simulink model "dynamicANN"  (R2019b)
settings: Solver=VariableStepAuto  StartTime=0.0  StopTime=5  RelTol=1e-3
values from neighbouring files (symbols this model uses):
  a = 87.548e-3    (= 0.087548)    [main.m]
  b = 132.452e-3    (= 0.132452)    [main.m]
  d = 22.452e-3    (= 0.022452)    [main.m]
  delta = [dX 0 0 0; -dX 0 0 0; 0 dXdot 0 0; 0 -dXdot 0 0; 0 0 dY 0; 0 0 -dY 0; 0 0 0 dYdot; 0 0 0 -dYdot]    [dyn_coeff.m]    (also in main.m = 2.5e-05)
  F1 = mass*g-F2    (= 22.4020462598)    [main.m]
  F2 = a*mass*g/(a+b)    (= 14.8072837402)    [main.m]
  g = 9.8    [EOM.m]    (also in main.m = 9.81)
  Jd = 0.047331604    [main.m]
  Jp = 0.00075    [main.m]
  Kps = (Vmax-Vmin)/(Hmax-Hmin)    (= 1666.66666667)    [main.m]
  Ksv = 30    [main.m]
  mass = 3.793    [main.m]
  omega = operational_parameters(1)*2*pi/60    [CalculateLoadCapacity.m]    (also in main.m = 146.607657168)
  s = 30e-3    (= 0.03)    [main.m]    (also in nntrainingsetgen.m = size(XC))
  tau = 0.12    [main.m]
  taus = 0.00125    [main.m]
  Ts = 1/fs    (= 0.001)    [main.m]
libraries: neural x424, simulink x2
(part 8 of 10)

== system dynamicANN/ROTOR SYSTEM WITH ANN/B1NN/Layer 2/Delays 1 ==
  "p{2}" : Inport  PortDimensions=100
      mask Display: e = 0.06;c1 = [120 230 180]/255;c2 = ([120 230 180]+0)/(256+128);c3 = ([120 230 180]+128)/(256+128);patch([0 1 1 0],[0 0 1 1],c1);patch([0 1 1 1-e 1-e 0+e],[0 0 1 1-e 0+e 0+e],c2);patch([0 0 1 1-e 0+e 0+e],[0 1 1 1-e 1-e 0+e],c3);plot([0 1 1 0 0],[0 0 1 1 0]);
  mux : Mux  Inputs=1
      mask Display: e = 0.06;c1 = [120 150 230]/255;c2 = ([120 150 230]+0)/383;c3 = ([120 150 230]+128)/383;patch([0 1 1 0],[0 0 1 1],c1);patch([0 1 1 1-e 1-e 0+e],[0 0 1 1-e 0+e 0+e],c2);patch([0 0 1 1-e 0+e 0+e],[0 1 1 1-e 1-e 0+e],c3);plot([0 1 1 0 0],[0 0 1 1 0]);disp('Mux')
  "pd{2,1}" : Outport
      mask Display: e = 0.06;c1 = [120 230 180]/255;c2 = ([120 230 180]+0)/(256+128);c3 = ([120 230 180]+128)/(256+128);patch([0 1 1 0],[0 0 1 1],c1);patch([0 1 1 1-e 1-e 0+e],[0 0 1 1-e 0+e 0+e],c2);patch([0 0 1 1-e 0+e 0+e],[0 1 1 1-e 1-e 0+e],c3);plot([0 1 1 0 0],[0 0 1 1 0]);
  wires:
  "p{2}"/1 -> mux/1
  mux/1 -> "pd{2,1}"/1

== system dynamicANN/ROTOR SYSTEM WITH ANN/B1NN/Layer 2/LW{2,1} ==
  "ad{2,1}" : Inport  PortDimensions=100
      mask Display: e = 0.06;c1 = [120 230 180]/255;c2 = ([120 230 180]+0)/(256+128);c3 = ([120 230 180]+128)/(256+128);patch([0 1 1 0],[0 0 1 1],c1);patch([0 1 1 1-e 1-e 0+e],[0 0 1 1-e 0+e 0+e],c2);patch([0 0 1 1-e 0+e 0+e],[0 1 1 1-e 1-e 0+e],c3);plot([0 1 1 0 0],[0 0 1 1 0]);
  "IW{2,1}(1,:)'" : Constant  Value=[-4.30818797311500389923821785487234592437744140625;0.1752068552208518037449636040037148632109165191650390625;1.6512760960076289240561209226143546402454376220703125;-1.2668488416247047911866729918983764946460723876953125;-0.169916708135180172245526364349643699824810028076171875;2.667525323070837117711562314070761203765869140625;-3.694593268415584663699746670317836105823516845703125;-0.194624707793134177347127433677087537944316864013671875;3.883534816499157660274477166240103542804718017578125;-4.8924351217341808251148904673755168914794921875;0.16008181045926705987625382476835511624813079833984375;-4.0208522454679798130428025615401566028594970703125;2.81348078614510210826438196818344295024871826171875;-0.09088682268917881723613305666731321252882480621337890625;-0.361803208282506283399726498828385956585407257080078125;-2.550539713092682791995002844487316906452178955078125;0.06642984533116191858681531812180764973163604736328125;4.87354419159413776441169829922728240489959716796875;-3.155434137388119619771487123216502368450164794921875;0.04540205268647821978955647637121728621423244476318359375;3.523762597164889154299771689693443477153778076171875;1.2480467061721984833866372355259954929351806640625;-2.496517162071746565032981379772536456584930419921875;1.5074739853906506947822663278202526271343231201171875;-1.117099106699883659388206069706939160823822021484375;-1.7985864180199346851196651186910457909107208251953125;-0.56163748275957170452699074303382076323032379150390625;-1.8836310342766171554984566682833246886730194091796875;0.30990689097744639202147709511336870491504669189453125;-1.0077815603465609672895197945763356983661651611328125;3.362573325147230729470493315602652728557586669921875;2.008823959936939740344996607745997607707977294921875;-0.636176137703270416778877915930934250354766845703125;0.313469372433028359292705999905592761933803558349609375;0.248267474312885372267345474028843455016613006591796875;0.210498516029080484646129889370058663189411163330078125;-0.338835866719135847535682160014403052628040313720703125;0.62947316963917743226630818753619678318500518798828125;3.454920994847224147150654971483163535594940185546875;4.953382971499575404550341772846877574920654296875;0.93530825830339858750761550254537723958492279052734375;1.252326977859621326416572628659196197986602783203125;0.051711000248056804284857435050071217119693756103515625;0.035047972353667071476746031066795694641768932342529296875;3.121997848768389705043091453262604773044586181640625;-0.62693281706946824005655116707202978432178497314453125;-7.53168886405034410103098707622848451137542724609375;2.8258369473664828319670050404965877532958984375;-3.5103810578844019119060249067842960357666015625;0.54822400418842265334973262724815867841243743896484375;-3.6507498536171620884260846651159226894378662109375;-2.838093873507663289501579129137098789215087890625;-0.1063584286302850234751105062969145365059375762939453125;2.71882444674755152647094291751272976398468017578125;-0.90305330807928718694910230624373070895671844482421875;-2.9292466026121370958890111069194972515106201171875;0.09624910207705629494601140550003037787973880767822265625;-6.25458905085562744119442868395708501338958740234375;0.93057375925756591339421675002085976302623748779296875;4.3108234020723816826148322434164583683013916015625;0.877335859031184828182858836953528225421905517578125;0.62320080161543012220448645166470669209957122802734375;2.5020205204075214311387753696180880069732666015625;3.044774500165214448088590870611369609832763671875;2.49364090933709547925900551490485668182373046875;4.06208905541347586876099740038625895977020263671875;0.352402568009233918555622722124098800122737884521484375;-2.179626460191489645268347885576076805591583251953125;-1.6720918879663491107834261129028163850307464599609375;-0.174128156259417465889782761223614215850830078125;-1.0133234558063615171619176180684007704257965087890625;-0.87954323399977429875917778190341778099536895751953125 ...(+1546 chars)]
      mask Display: e = 0.06;c1 = [120 150 230]/255;c2 = ([120 150 230]+0)/383;c3 = ([120 150 230]+128)/383;patch([0 1 1 0],[0 0 1 1],c1);patch([0 1 1 1-e 1-e 0+e],[0 0 1 1-e 0+e 0+e],c2);patch([0 0 1 1-e 0+e 0+e],[0 1 1 1-e 1-e 0+e],c3);plot([0 1 1 0 0],[0 0 1 1 0]);disp('weights');
  "IW{2,1}(2,:)'" : Constant  Value=[-5.19148173001544233073900613817386329174041748046875;1.40690786182195726183863371261395514011383056640625;-0.30464941675884082972203259487287141382694244384765625;-2.90594055753510804862571603734977543354034423828125;-5.2786442959257211526846731430850923061370849609375;-4.749610968610955552549057756550610065460205078125;2.000959904419529866714810850680805742740631103515625;0.958774635589488166687033299240283668041229248046875;-1.51433580109468568508646058035083115100860595703125;3.012127212742239379394959541969001293182373046875;2.030557542334976428577419937937520444393157958984375;5.1979119527008545986745957634411752223968505859375;-2.63344015879183235284699549083597958087921142578125;1.595792101490900449789478443562984466552734375;3.606400898368459451148737571202218532562255859375;-3.562582906379017533282649310422129929065704345703125;0.377198036894335120283727746937074698507785797119140625;-5.36845758424446817258512965054251253604888916015625;1.749142625921928040355624034418724477291107177734375;-2.048149223373259442126936846761964261531829833984375;1.004846893971668375655781346722505986690521240234375;5.509896229123445010600335081107914447784423828125;-1.17397493449301304480059116031043231487274169921875;2.565644301520971115593283684574998915195465087890625;1.48695237349638631485504447482526302337646484375;5.33739042575180011596103213378228247165679931640625;-4.04781195330859500103315440355800092220306396484375;-4.03609609549113290682953447685576975345611572265625;-3.27872494454356999682431705878116190433502197265625;5.2623832468193398881339817307889461517333984375;-1.0030830173197851085120646530413068830966949462890625;-1.71802080792238331952148655545897781848907470703125;6.68822525979784554550633401959203183650970458984375;2.0864430844354320271349934046156704425811767578125;1.562852599531094455187485436908900737762451171875;1.5064184874930803825776592930196784436702728271484375;2.740713679439760408484971776488237082958221435546875;-1.895606311298295931777602163492701947689056396484375;-0.09516882270704461743715540933408192358911037445068359375;1.3456293400895000811345880720182321965694427490234375;5.0750660913960015108159495866857469081878662109375;2.233404782953354317243110926938243210315704345703125;-2.14084605198024036099013756029307842254638671875;-0.0019595480400120247020667729742626761435531079769134521484375;-4.2725650308945670730054189334623515605926513671875;0.87412801328391698252318064987775869667530059814453125;0.047472919180466109645433192554264678619801998138427734375;-5.06606359435499609134012644062750041484832763671875;-0.06682069419569010293447064441352267749607563018798828125;-0.09793427088049301565408910619225935079157352447509765625;-1.0419264279899722591693489448516629636287689208984375;0.61485468084976802050078958927770145237445831298828125;-0.10281300772583672198390303265114198438823223114013671875;0.0295657560599492837127844069300408591516315937042236328125;-4.45784329010434543505425608600489795207977294921875;-8.89392354954583197468309663236141204833984375;1.298006282970192604153680804301984608173370361328125;1.54614271746198905788105548708699643611907958984375;4.3170427254455372434449600405059754848480224609375;6.17411702636139825273176029440946877002716064453125;-2.5270013527782300144508553785271942615509033203125;6.74658722376797381770074935047887265682220458984375;-6.30276208841053975362456185393966734409332275390625;-0.40027132066036752444659896355005912482738494873046875;0.394702758514758389463139565123128704726696014404296875;-3.743958856611741214948096967418678104877471923828125;3.8121019710154513404631870798766613006591796875;1.2196396694109121749960422675940208137035369873046875;-3.265314950442772090610787927289493381977081298828125;-0.73557517790217541442387982897344045341014862060546875;1.34049068929635684099821446579881012439727783203125;-5.658636280675874985490736435167491436004638671875;2.19036079829303798049977558548562228679656982421875 ...(+1476 chars)]
      mask Display: e = 0.06;c1 = [120 150 230]/255;c2 = ([120 150 230]+0)/383;c3 = ([120 150 230]+128)/383;patch([0 1 1 0],[0 0 1 1],c1);patch([0 1 1 1-e 1-e 0+e],[0 0 1 1-e 0+e 0+e],c2);patch([0 0 1 1-e 0+e 0+e],[0 1 1 1-e 1-e 0+e],c3);plot([0 1 1 0 0],[0 0 1 1 0]);disp('weights');
  Mux : Mux  Inputs=2
      mask Display: e = 0.06;c1 = [120 150 230]/255;c2 = ([120 150 230]+0)/383;c3 = ([120 150 230]+128)/383;patch([0 1 1 0],[0 0 1 1],c1);patch([0 1 1 1-e 1-e 0+e],[0 0 1 1-e 0+e 0+e],c2);patch([0 0 1 1-e 0+e 0+e],[0 1 1 1-e 1-e 0+e],c3);plot([0 1 1 0 0],[0 0 1 1 0]);disp('Mux');
  dotprod1 : neural/Weight Functions/dotprod
      settings: SourceProductName=Deep Learning Toolbox
  dotprod2 : neural/Weight Functions/dotprod
      settings: SourceProductName=Deep Learning Toolbox
  "lz{2,1}" : Outport
      mask Display: e = 0.06;c1 = [120 230 180]/255;c2 = ([120 230 180]+0)/(256+128);c3 = ([120 230 180]+128)/(256+128);patch([0 1 1 0],[0 0 1 1],c1);patch([0 1 1 1-e 1-e 0+e],[0 0 1 1-e 0+e 0+e],c2);patch([0 0 1 1-e 0+e 0+e],[0 1 1 1-e 1-e 0+e],c3);plot([0 1 1 0 0],[0 0 1 1 0]);
  wires:
  "IW{2,1}(1,:)'"/1 -> dotprod1/1
  "ad{2,1}"/1 -> dotprod1/2, dotprod2/2
  dotprod1/1 -> Mux/1
  "IW{2,1}(2,:)'"/1 -> dotprod2/1
  dotprod2/1 -> Mux/2
  Mux/1 -> "lz{2,1}"/1

== system dynamicANN/ROTOR SYSTEM WITH ANN/B2NN/Layer 1/Delays 1 ==
  "p{1}" : Inport  PortDimensions=4
      mask Display: e = 0.06;c1 = [120 230 180]/255;c2 = ([120 230 180]+0)/(256+128);c3 = ([120 230 180]+128)/(256+128);patch([0 1 1 0],[0 0 1 1],c1);patch([0 1 1 1-e 1-e 0+e],[0 0 1 1-e 0+e 0+e],c2);patch([0 0 1 1-e 0+e 0+e],[0 1 1 1-e 1-e 0+e],c3);plot([0 1 1 0 0],[0 0 1 1 0]);
  mux : Mux  Inputs=1
      mask Display: e = 0.06;c1 = [120 150 230]/255;c2 = ([120 150 230]+0)/383;c3 = ([120 150 230]+128)/383;patch([0 1 1 0],[0 0 1 1],c1);patch([0 1 1 1-e 1-e 0+e],[0 0 1 1-e 0+e 0+e],c2);patch([0 0 1 1-e 0+e 0+e],[0 1 1 1-e 1-e 0+e],c3);plot([0 1 1 0 0],[0 0 1 1 0]);disp('Mux')
  "pd{1,1}" : Outport
      mask Display: e = 0.06;c1 = [120 230 180]/255;c2 = ([120 230 180]+0)/(256+128);c3 = ([120 230 180]+128)/(256+128);patch([0 1 1 0],[0 0 1 1],c1);patch([0 1 1 1-e 1-e 0+e],[0 0 1 1-e 0+e 0+e],c2);patch([0 0 1 1-e 0+e 0+e],[0 1 1 1-e 1-e 0+e],c3);plot([0 1 1 0 0],[0 0 1 1 0]);
  wires:
  "p{1}"/1 -> mux/1
  mux/1 -> "pd{1,1}"/1
